simulink model "drone_PID_1126"  (R2021a)
settings: Solver=FixedStepAuto  StartTime=0.0  StopTime=10.0  RelTol=1e-3  EnableMultiTasking=on
model workspace (MAT data in the model file):
  H_G = 2
  Sv = 1300
  Ta = 4000
  Tb = 1600
  Ts = 0.016
  VOL_center = 1515
  V_G = 100
  step_R = 0.2
  volume_G = 100
undefined symbols (not defined in the file or in its folder): AUX, dev, pwm_output1
libraries: px4Sensorslib x8, cstblocks x4, px4lib x4, simulink x1, px4uORBlib x1
settings Model: ExtModeTrigDuration=10  Creator=Kawaguchi  LastModifiedBy=beket
settings SolverCC: PositivePriorityOrder=on
settings OptimizationCC: EnhancedBackFolding=on  PassReuseOutputArgsAs=Individual arguments  ZeroExternalMemoryAtStartup=off  ZeroInternalMemoryAtStartup=off  MaxStackSize=64  OptimizeBlockOrder=speed  DifferentSizesBufferReuse=on  OptimizationCustomize=off  EfficientTunableParamExpr=on
settings DebuggingCC: ParameterTunabilityLossMsg=error
settings HardwareCC: ProdBitPerPointer=32  ProdBitPerSizeT=32  ProdBitPerPtrDiffT=32  ProdLargestAtomicInteger=Long  ProdLargestAtomicFloat=Double  ProdWordSize=32  ProdLongLongMode=on  ProdHWDeviceType=ARM Compatible->ARM Cortex
settings SFSimCC: MATLABDynamicMemAlloc=off  SimTargetLang=C++
settings RTWCC: SystemTargetFile=ert.tlc  HardwareBoard=PX4 Pixhawk 4  TLCOptions="-aInlineSetEventsForThisBaseRateFcn=TLC_FALSE -aSuppressMultiTaskScheduler=TLC_FALSE  -aRateBasedStepFcn=0"  TemplateMakefile=ert_default_tmf  Toolchain=GNU Tools for PX4 Autopilots  TargetLang=C++
settings CodeAppCC: ForceParamTrailComments=on  IgnoreCustomStorageClasses=off  OperatorAnnotations=on  SimulinkDataObjDesc=on  SFDataObjDesc=on  InsertBlockDesc=on
settings ERTTargetCC: ExtModeTransport=3  ExtModeStaticAlloc=on  ExtModeStaticAllocSize=1024  ExtModeMexFile=ext_xcp  ExtModeIntrfLevel=Level2 - Open

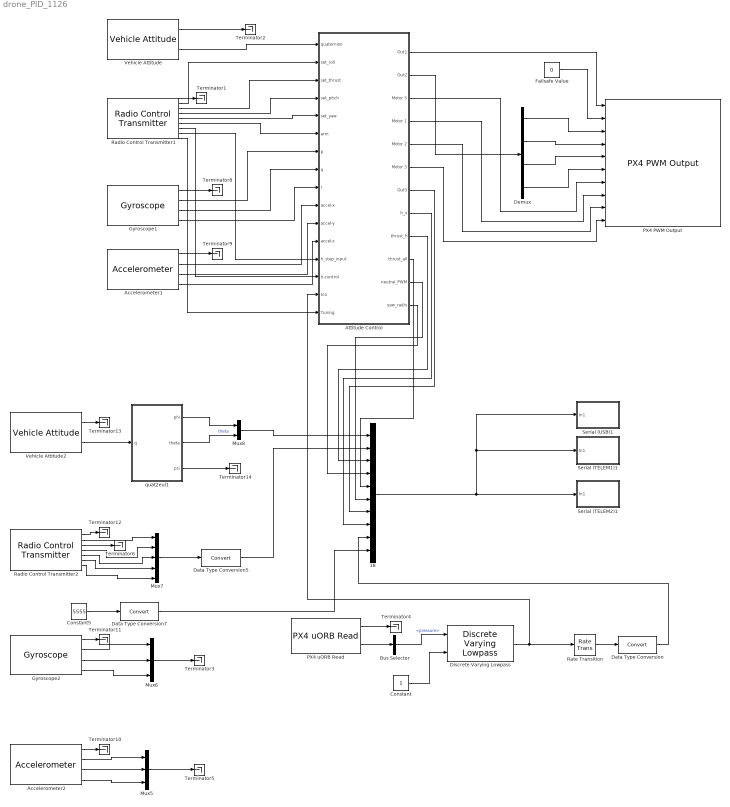
== system drone_PID_1126 ==
  18 : Mux  Inputs=10
  Accelerometer1 : px4Sensorslib/Accelerometer  uorbTimeStamp=off  BlockingMode=off  BlockTimeout=1e-3  sampleTime=1/250
      settings: SourceProductBaseCode=PX4AUTOPILOTS
  Accelerometer2 : px4Sensorslib/Accelerometer  uorbTimeStamp=off  BlockingMode=off  BlockTimeout=1e-3  sampleTime=Ts
      settings: SourceProductBaseCode=PX4AUTOPILOTS
  Attitude Control : Subsystem
  Bus Selector : BusSelector  OutputSignals=pressure
  Constant : Constant
  Constant5 : Constant  Value=5555
  Data Type Conversion : DataTypeConversion
  Data Type Conversion5 : DataTypeConversion
  Data Type Conversion7 : DataTypeConversion
  Demux : Demux
  Discrete Varying Lowpass : cstblocks/Linear Parameter Varying/Discrete Varying Lowpass  N=1  w0=0  Ts=1/250
      settings: SourceProductBaseCode=CT
  Failsafe Value : Constant  Value=0  OutDataTypeStr=boolean  SampleTime=-1
  Gyroscope1 : px4Sensorslib/Gyroscope  uorbTimeStamp=off  BlockingMode=off  BlockTimeout=1e-3  sampleTime=1/250
      settings: SourceProductBaseCode=PX4AUTOPILOTS
  Gyroscope2 : px4Sensorslib/Gyroscope  uorbTimeStamp=off  BlockingMode=off  BlockTimeout=1e-3  sampleTime=Ts
      settings: SourceProductBaseCode=PX4AUTOPILOTS
  Mux5 : Mux  Inputs=3
  Mux6 : Mux  Inputs=3
  Mux7 : Mux  Inputs=5
  Mux8 : Mux  Inputs=2
  PX4 PWM Output : px4lib/PX4 PWM Output  pwmDevice=AUX (/dev/pwm_output1)  pwmChannel1_=on  pwmChannel2_=on  pwmChannel3_=on  pwmChannel4_=on  pwmChannel5_=on  pwmChannel6_=on  pwmChannel7_=on  pwmChannel8_=on  forceTerminateFailsafe=off  outputErrorStatus=off
      settings: SourceProductBaseCode=PX4AUTOPILOTS
  PX4 uORB Read : px4uORBlib/PX4 uORB Read  uORBTopic=sensor_baro  selectInstance=sensor_baro  SampleTime=1/250  BlockingMode=off  BlockTimeout=1e-3
      settings: SourceProductBaseCode=PX4AUTOPILOTS
  Radio Control Transmitter1 : px4Sensorslib/Radio Control Transmitter  channel1=on  channel2=on  channel3=on  channel4=on  channel5=on  channel6=on  channel7=on  channel8=on  channel_count=off  rssi=off  rc_input_source=off  timestamp_last_signal=off  time_stamp=off  sampleTime=1/250  BlockingMode=off  BlockTimeout=5
      settings: SourceProductBaseCode=PX4AUTOPILOTS
  Radio Control Transmitter2 : px4Sensorslib/Radio Control Transmitter  channel1=on  channel2=on  channel3=on  channel4=on  channel5=on  channel6=off  channel7=on  channel8=off  channel_count=off  rssi=off  rc_input_source=off  timestamp_last_signal=off  time_stamp=off  sampleTime=Ts  BlockingMode=off  BlockTimeout=5
      settings: SourceProductBaseCode=PX4AUTOPILOTS
  Rate Transition : RateTransition  OutPortSampleTimeOpt=Multiple of input port sample time  OutPortSampleTimeMultiple=4  OutPortSampleTime=4
  Serial (TELEM1)1 : Subsystem
  Serial (TELEM2)1 : Subsystem
  Serial (USB)1 : Subsystem
  Terminator{1..6,8..14} (13 alike) : Terminator
  Vehicle Attitude : px4Sensorslib/Vehicle Attitude  rollRate=off  pitchRate=off  yawRate=off  quaternion=on  uorbTimeStamp=off  BlockingMode=off  BlockTimeout=0.001  sampleTime=1/250
      settings: SourceProductBaseCode=PX4AUTOPILOTS
  Vehicle Attitude2 : px4Sensorslib/Vehicle Attitude  rollRate=off  pitchRate=off  yawRate=off  quaternion=on  uorbTimeStamp=off  BlockingMode=off  BlockTimeout=0.001  sampleTime=Ts
      settings: SourceProductBaseCode=PX4AUTOPILOTS
  quat2eul1 : MATLAB Function  TreatAsAtomicUnit=on
  wires:
  Vehicle Attitude/1 -> Terminator2/1
  Vehicle Attitude/2 -> Attitude Control/1(quaternion)
  Radio Control Transmitter1/1 -> Terminator1/1
  Radio Control Transmitter1/2 -> Attitude Control/2(set_roll)
  Radio Control Transmitter1/3 -> Attitude Control/3(set_thrust)
  Radio Control Transmitter1/4 -> Attitude Control/4(set_pitch)
  Radio Control Transmitter1/5 -> Attitude Control/5(set_yaw)
  Radio Control Transmitter1/6 -> Attitude Control/6(arm)
  Accelerometer1/1 -> Terminator9/1
  Gyroscope1/1 -> Terminator8/1
  Gyroscope1/2 -> Attitude Control/7(p)
  Gyroscope1/3 -> Attitude Control/8(q)
  Gyroscope1/4 -> Attitude Control/9(r)
  Accelerometer1/2 -> Attitude Control/10(accel-x)
  Accelerometer1/3 -> Attitude Control/11(accel-y)
  Accelerometer1/4 -> Attitude Control/12(accel-z)
  Data Type Conversion7/1 -> 18/10
  Accelerometer2/4 -> Mux5/3
  quat2eul1/2(theta) -> Mux8/2  "theta"
  Radio Control Transmitter2/4 -> Mux7/2
  Mux7/1 -> Data Type Conversion5/1
  18/1 -> Serial (TELEM1)1/1(In1), Serial (USB)1/1(In1), Serial (TELEM2)1/1(In1)
  Gyroscope2/4 -> Mux6/3
  quat2eul1/1(phi) -> Mux8/1
  Radio Control Transmitter2/1 -> Terminator12/1
  Gyroscope2/1 -> Terminator11/1
  Accelerometer2/3 -> Mux5/2
  Constant5/1 -> Data Type Conversion7/1
  Accelerometer2/2 -> Mux5/1
  Radio Control Transmitter2/3 -> Terminator6/1
  Accelerometer2/1 -> Terminator10/1
  Vehicle Attitude2/1 -> Terminator13/1
  Radio Control Transmitter2/2 -> Mux7/1
  Gyroscope2/3 -> Mux6/2
  quat2eul1/3(psi) -> Terminator14/1
  Gyroscope2/2 -> Mux6/1
  Vehicle Attitude2/2 -> quat2eul1/1(q)
  Mux8/1 -> 18/1
  Data Type Conversion5/1 -> 18/2
  Mux5/1 -> Terminator5/1
  Attitude Control/1(Out1) -> PX4 PWM Output/1
  Demux/1 -> PX4 PWM Output/3
  Demux/2 -> PX4 PWM Output/4
  Demux/3 -> PX4 PWM Output/5
  Demux/4 -> PX4 PWM Output/6
  Failsafe Value/1 -> PX4 PWM Output/2
  Attitude Control/3(Motor 5) -> PX4 PWM Output/7
  Attitude Control/4(Motor 1) -> PX4 PWM Output/8
  Attitude Control/5(Motor 2) -> PX4 PWM Output/9
  Attitude Control/6(Motor 3) -> PX4 PWM Output/10
  Radio Control Transmitter2/5 -> Mux7/3
  Attitude Control/7(Out3) -> 18/7
  Mux6/1 -> Terminator3/1
  Radio Control Transmitter2/6 -> Mux7/4
  PX4 uORB Read/1 -> Terminator4/1
  PX4 uORB Read/2 -> Bus Selector/1
  Bus Selector/1 -> Discrete Varying Lowpass/1  "<pressure>"
  Data Type Conversion/1 -> 18/9
  Discrete Varying Lowpass/1 -> Rate Transition/1, Attitude Control/15(In1)
  Constant/1 -> Discrete Varying Lowpass/2
  Radio Control Transmitter2/7 -> Mux7/5
  Radio Control Transmitter1/8 -> Attitude Control/13(h_step_input)
  Radio Control Transmitter1/7 -> Attitude Control/14(h-control)
  Rate Transition/1 -> Data Type Conversion/1
  Radio Control Transmitter1/9 -> Attitude Control/16(Tuning)
  Attitude Control/8(h_x) -> 18/8
  Attitude Control/2(Out2) -> Demux/1
  Attitude Control/9(thrust_h) -> 18/3
  Attitude Control/12(yaw_rad/s) -> 18/4
  Attitude Control/10(thrust_all) -> 18/5
  Attitude Control/11(neutral_PWM) -> 18/6

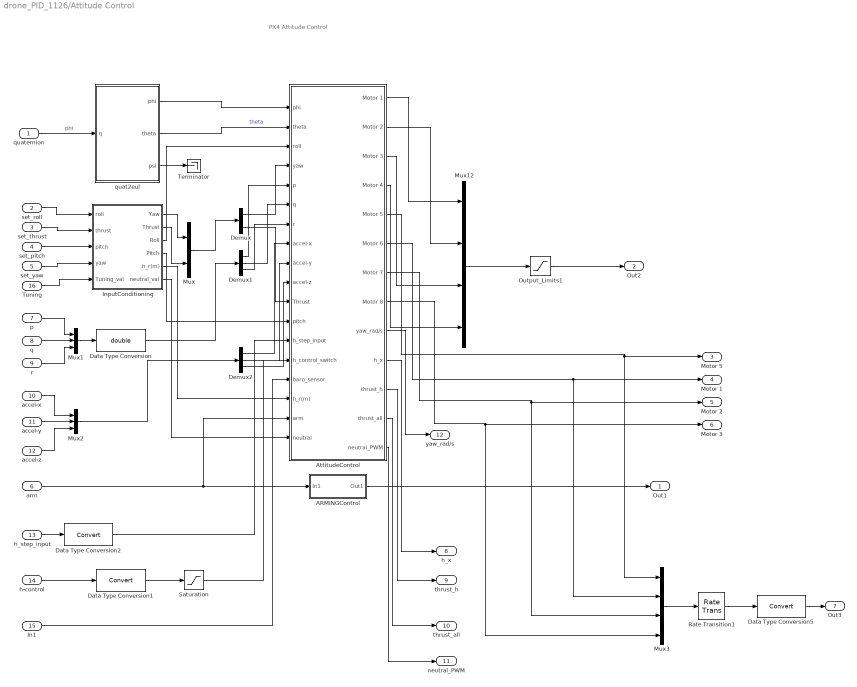
== system drone_PID_1126/Attitude Control ==
  note: PX4 Attitude Control
  quaternion : Inport
  set_roll : Inport  Port=2  OutDataTypeStr=uint16
  set_thrust : Inport  Port=3  OutDataTypeStr=uint16
  set_pitch : Inport  Port=4  OutDataTypeStr=uint16
  set_yaw : Inport  Port=5  OutDataTypeStr=uint16
  arm : Inport  Port=6  OutDataTypeStr=uint16
  p : Inport  Port=7
  q : Inport  Port=8
  r : Inport  Port=9
  accel-x : Inport  Port=10
  accel-y : Inport  Port=11
  accel-z : Inport  Port=12
  h_step_input : Inport  Port=13
  h-control : Inport  Port=14
  In1 : Inport  Port=15
  Tuning : Inport  Port=16
  ARMINGControl : Subsystem
  AttitudeControl : Subsystem
  Data Type Conversion : DataTypeConversion  OutDataTypeStr=double
  Data Type Conversion1 : DataTypeConversion
  Data Type Conversion2 : DataTypeConversion
  Data Type Conversion5 : DataTypeConversion
  Demux : Demux  Outputs=2
  Demux1 : Demux  Outputs=3
  Demux2 : Demux  Outputs=3
  InputConditioning : Subsystem
  Mux : Mux  Inputs=2
  Mux1 : Mux  Inputs=3
  Mux12 : Mux
  Mux2 : Mux  Inputs=3
  Mux3 : Mux
  Output_Limits1 : Saturate  UpperLimit=2000  LowerLimit=1000
  Rate Transition1 : RateTransition  OutPortSampleTimeOpt=Multiple of input port sample time  OutPortSampleTimeMultiple=4
  Saturation : Saturate  UpperLimit=1600  LowerLimit=0
  Terminator : Terminator
  quat2eul : MATLAB Function  TreatAsAtomicUnit=on
  Out1 : Outport  VectorParamsAs1DForOutWhenUnconnected=off
  Out2 : Outport  Port=2  VectorParamsAs1DForOutWhenUnconnected=off
  Motor 5 : Outport  Port=3  OutDataTypeStr=uint16  VectorParamsAs1DForOutWhenUnconnected=off
  Motor 1 : Outport  Port=4  OutDataTypeStr=uint16  VectorParamsAs1DForOutWhenUnconnected=off
  Motor 2 : Outport  Port=5  OutDataTypeStr=uint16  VectorParamsAs1DForOutWhenUnconnected=off
  Motor 3 : Outport  Port=6  OutDataTypeStr=uint16  VectorParamsAs1DForOutWhenUnconnected=off
  Out3 : Outport  Port=7
  h_x : Outport  Port=8
  thrust_h : Outport  Port=9
  thrust_all : Outport  Port=10
  neutral_PWM : Outport  Port=11
  yaw_rad/s : Outport  Port=12
  wires:
  set_roll/1 -> InputConditioning/1(roll)
  arm/1 -> AttitudeControl/17(arm), ARMINGControl/1(In1)
  quat2eul/2(theta) -> AttitudeControl/2(theta)  "theta"
  Output_Limits1/1 -> Out2/1
  Mux12/1 -> Output_Limits1/1
  ARMINGControl/1(Out1) -> Out1/1
  set_yaw/1 -> InputConditioning/4(yaw)
  quaternion/1 -> quat2eul/1(q)  "phi"
  quat2eul/1(phi) -> AttitudeControl/1(phi)
  quat2eul/3(psi) -> Terminator/1
  AttitudeControl/1(Motor 1) -> Mux12/1
  AttitudeControl/2(Motor 2) -> Mux12/2
  AttitudeControl/3(Motor 3) -> Mux12/3
  AttitudeControl/4(Motor 4) -> Mux12/4
  Mux/1 -> Demux/1
  p/1 -> Mux1/1
  r/1 -> Mux1/3
  Mux1/1 -> Data Type Conversion/1
  Demux1/2 -> AttitudeControl/6(q)
  Demux1/1 -> AttitudeControl/5(p)
  Demux1/3 -> AttitudeControl/7(r)
  accel-y/1 -> Mux2/2
  accel-x/1 -> Mux2/1
  accel-z/1 -> Mux2/3
  Mux2/1 -> Demux2/1
  Demux2/2 -> AttitudeControl/9(accel-y)
  Demux2/1 -> AttitudeControl/8(accel-x)
  Demux2/3 -> AttitudeControl/10(accel-z)
  InputConditioning/1(Yaw) -> Mux/1
  InputConditioning/2(Thrust) -> Mux/2
  Demux/1 -> AttitudeControl/4(yaw)
  Demux/2 -> AttitudeControl/11(Thrust)
  InputConditioning/3(Roll) -> AttitudeControl/3(roll)
  InputConditioning/4(Pitch) -> AttitudeControl/12(pitch)
  set_thrust/1 -> InputConditioning/2(thrust)
  set_pitch/1 -> InputConditioning/3(pitch)
  q/1 -> Mux1/2
  Data Type Conversion/1 -> Demux1/1
  AttitudeControl/5(Motor 5) -> Mux3/1, Motor 5/1
  AttitudeControl/8(Motor 8) -> Mux3/4, Motor 3/1
  AttitudeControl/7(Motor 7) -> Mux3/3, Motor 2/1
  AttitudeControl/6(Motor 6) -> Mux3/2, Motor 1/1
  Mux3/1 -> Rate Transition1/1
  Data Type Conversion5/1 -> Out3/1
  Rate Transition1/1 -> Data Type Conversion5/1
  AttitudeControl/9(yaw_rad/s) -> yaw_rad/s/1
  h_step_input/1 -> Data Type Conversion2/1
  Data Type Conversion2/1 -> AttitudeControl/13(h_step_input)
  h-control/1 -> Data Type Conversion1/1
  Data Type Conversion1/1 -> Saturation/1
  In1/1 -> AttitudeControl/15(baro_sensor)
  AttitudeControl/10(h_x) -> h_x/1
  InputConditioning/5(h_r(m)) -> AttitudeControl/16(h_r(m))
  Tuning/1 -> InputConditioning/5(Tuning_val)
  InputConditioning/6(neutral_val) -> AttitudeControl/18(neutral)
  Saturation/1 -> AttitudeControl/14(h_control_switch)
  AttitudeControl/11(thrust_h) -> thrust_h/1
  AttitudeControl/12(thrust_all) -> thrust_all/1
  AttitudeControl/13(neutral_PWM) -> neutral_PWM/1

== system drone_PID_1126/Serial (TELEM1)1 ==
  In1 : Inport
  Cast To Single1 : DataTypeConversion  OutDataTypeStr=single
  Serial Transmit1 : px4lib/Serial Transmit  SCIModule=/dev/ttyS1
      settings: SourceProductBaseCode=PX4AUTOPILOTS
  wires:
  Cast To Single1/1 -> Serial Transmit1/1
  In1/1 -> Cast To Single1/1

== system drone_PID_1126/Serial (TELEM2)1 ==
  In1 : Inport
  Cast To Single1 : DataTypeConversion  OutDataTypeStr=single
  Serial Transmit1 : px4lib/Serial Transmit  SCIModule=/dev/ttyS2
      settings: SourceProductBaseCode=PX4AUTOPILOTS
  wires:
  Cast To Single1/1 -> Serial Transmit1/1
  In1/1 -> Cast To Single1/1

== system drone_PID_1126/Serial (USB)1 ==
  In1 : Inport
  Cast To Single1 : DataTypeConversion  OutDataTypeStr=single
  Serial Transmit1 : px4lib/Serial Transmit  SCIModule=/dev/ttyACM0
      settings: SourceProductBaseCode=PX4AUTOPILOTS
  wires:
  Cast To Single1/1 -> Serial Transmit1/1
  In1/1 -> Cast To Single1/1

== system drone_PID_1126/Attitude Control/ARMINGControl ==
  In1 : Inport
  Compare To Constant3 : simulink/Logic and Bit Operations/Compare To Constant  relop=>=  const=uint16(1500)  OutDataTypeStr=boolean
  Out1 : Outport  VectorParamsAs1DForOutWhenUnconnected=off
  wires:
  Compare To Constant3/1 -> Out1/1
  In1/1 -> Compare To Constant3/1

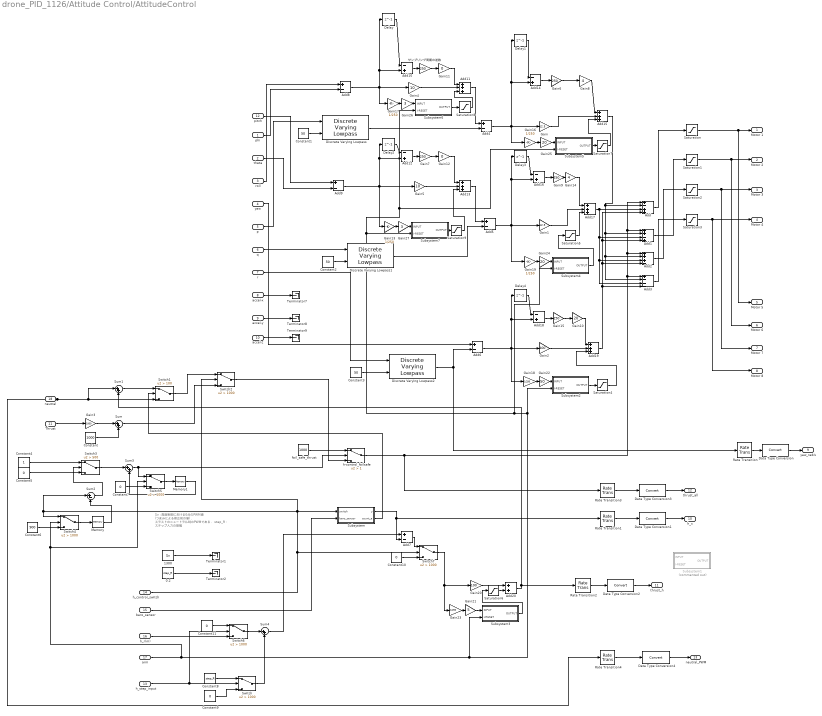
== system drone_PID_1126/Attitude Control/AttitudeControl ==
  note: Sv : 高度制御における0点のPWM値
      | 	(つまみによる修正前の値)．
      | スラストのニュートラル時のPWMである．
      |
      | step_R : ステップ入力の振幅
  phi : Inport
  theta : Inport  Port=2
  roll : Inport  Port=3
  yaw : Inport  Port=4
  p : Inport  Port=5
  q : Inport  Port=6
  r : Inport  Port=7
  accel-x : Inport  Port=8
  accel-y : Inport  Port=9
  accel-z : Inport  Port=10
  Thrust : Inport  Port=11
  pitch : Inport  Port=12
  h_step_input : Inport  Port=13
  h_control_switch : Inport  Port=14
  baro_sensor : Inport  Port=15
  h_r(m) : Inport  Port=16
  arm : Inport  Port=17
  neutral : Inport  Port=18
  0.2 : Constant  Value=step_R
  1300 : Constant  Value=Sv
  Add : Sum  Inputs=+-++
  Add1 : Sum  Inputs=++-+
  Add{10,12,14,16,18} (5 alike) : Sum  Inputs=-+
  Add{11,13,15,17,19} (5 alike) : Sum  Inputs=+++
  Add2 : Sum  Inputs=+++-
  Add20 : Sum
  Add3 : Sum  Inputs=+---
  Add{4..9} (6 alike) : Sum  Inputs=+-
  Constant : Constant  Value=1000
  Constant1 : Constant  Value=50
  Constant{5,7,9..11} (5 alike) : Constant  Value=0
  Constant2 : Constant  Value=50
  Constant3 : Constant  Value=50
  Constant4 : Constant
  Constant6 : Constant  Value=900
  Constant8 : Constant  Value=step_R
  Data Type Conversion{,1..4} (5 alike) : DataTypeConversion
  Delay{,1..4} (5 alike) : Delay  DelayLength=1  InitialCondition=0
  Discrete Varying Lowpass : cstblocks/Linear Parameter Varying/Discrete Varying Lowpass  N=1  w0=0  Ts=1/250
      settings: SourceProductBaseCode=CT
  Discrete Varying Lowpass1 : cstblocks/Linear Parameter Varying/Discrete Varying Lowpass  N=1  w0=0  Ts=1/250
      settings: SourceProductBaseCode=CT
  Discrete Varying Lowpass2 : cstblocks/Linear Parameter Varying/Discrete Varying Lowpass  N=1  w0=0  Ts=1/250
      settings: SourceProductBaseCode=CT
  Gain : Gain  Gain=12.5
  Gain1 : Gain  Gain=12.5
  Gain10 : Gain  Gain=20
  Gain11 : Gain  Gain=0
  Gain12 : Gain  Gain=0
  Gain{13,16..19,23} (6 alike) : Gain  Gain=1/250
  Gain14 : Gain  Gain=4
  Gain{6..7,9,15} (4 alike) : Gain  Gain=250
  Gain2 : Gain  Gain=400
  Gain20 : Gain  Gain=100
  Gain21 : Gain  Gain=5
  Gain22 : Gain  Gain=50
  Gain24 : Gain  Gain=20
  Gain25 : Gain  Gain=20
  Gain26 : Gain  Gain=3
  Gain27 : Gain  Gain=3
  Gain3 : Gain  Gain=1000
  Gain4 : Gain  Gain=10
  Gain5 : Gain  Gain=10
  Gain8 : Gain  Gain=4
  Memory : Memory  InitialCondition=900  InheritSampleTime=on
  Memory1 : Memory  InheritSampleTime=on
  Rate Transition{,1..4} (5 alike) : RateTransition  OutPortSampleTimeOpt=Multiple of input port sample time  OutPortSampleTimeMultiple=4  OutPortSampleTime=4
  Saturation{,1..3} (4 alike) : Saturate  UpperLimit=2000  LowerLimit=1000  OutDataTypeStr=uint16
  Saturation{4..5,7..9} (5 alike) : Saturate  UpperLimit=100  LowerLimit=-100
  Saturation6 : Saturate  UpperLimit=50  LowerLimit=-50
  Subsystem : Subsystem
  Subsystem1 : Subsystem  Commented=on
  Subsystem2 : Subsystem
  Subsystem3 : Subsystem
  Subsystem4 : Subsystem
  Subsystem5 : Subsystem
  Subsystem6 : Subsystem
  Subsystem7 : Subsystem
  Sum{,1,3..4} (4 alike) : Sum  Inputs=|++
  Sum2 : Sum  Inputs=|+-
  Switch{,2,4..7} (6 alike) : Switch  Criteria=u2 > Threshold  Threshold=1000
  Switch1 : Switch  Criteria=u2 > Threshold  Threshold=100
  Switch3 : Switch  Criteria=u2 > Threshold  Threshold=500
  Terminator{1..2,7..9} (5 alike) : Terminator
  fail_safe_thrust : Constant  Value=1000
  h-control_failsafe : Switch  Criteria=u2 > Threshold  Threshold=1
  サンプリング周期の逆数 : Gain  Gain=250
  Motor 1 : Outport  OutDataTypeStr=uint16  VectorParamsAs1DForOutWhenUnconnected=off
  Motor 2 : Outport  Port=2  OutDataTypeStr=uint16  VectorParamsAs1DForOutWhenUnconnected=off
  Motor 3 : Outport  Port=3  OutDataTypeStr=uint16  VectorParamsAs1DForOutWhenUnconnected=off
  Motor 4 : Outport  Port=4  OutDataTypeStr=uint16  VectorParamsAs1DForOutWhenUnconnected=off
  Motor 5 : Outport  Port=5  OutDataTypeStr=uint16  SampleTime=1/250  VectorParamsAs1DForOutWhenUnconnected=off
  Motor 6 : Outport  Port=6  OutDataTypeStr=uint16  VectorParamsAs1DForOutWhenUnconnected=off
  Motor 7 : Outport  Port=7  OutDataTypeStr=uint16  VectorParamsAs1DForOutWhenUnconnected=off
  Motor 8 : Outport  Port=8  OutDataTypeStr=uint16  VectorParamsAs1DForOutWhenUnconnected=off
  yaw_rad/s : Outport  Port=9
  h_x : Outport  Port=10
  thrust_h : Outport  Port=11
  thrust_all : Outport  Port=12
  neutral_PWM : Outport  Port=13
  wires:
  Add2/1 -> Saturation2/1
  Gain/1 -> Add15/2
  Add17/1 -> Add2/3, Add3/3, Add1/3, Add/3
  Add18/1 -> Gain15/1
  Add13/1 -> Add5/1
  Add14/1 -> Gain6/1
  Gain15/1 -> Gain10/1
  Gain11/1 -> Add11/1
  Gain1/1 -> Add17/2
  theta/1 -> Add9/2
  Gain14/1 -> Add17/1
  Gain12/1 -> Add13/1
  Gain5/1 -> Add13/2
  Saturation/1 -> Motor 5/1, Motor 1/1
  r/1 -> Discrete Varying Lowpass2/1
  Gain9/1 -> Gain14/1
  Gain6/1 -> Gain8/1
  Gain7/1 -> Gain12/1
  Add19/1 -> Add2/4, Add1/4, Add/4, Add3/4
  Add15/1 -> Add/2, Add1/2, Add2/2, Add3/2
  Add16/1 -> Gain9/1
  accel-z/1 -> Terminator9/1
  Delay3/1 -> Add16/1
  Gain10/1 -> Add19/1
  Delay/1 -> Add10/1
  Gain4/1 -> Add11/2
  サンプリング周期の逆数/1 -> Gain11/1
  Delay4/1 -> Add18/1
  Delay2/1 -> Add12/1
  Add11/1 -> Add4/1
  Add12/1 -> Gain7/1
  accel-x/1 -> Terminator7/1
  Add3/1 -> Saturation3/1
  Gain2/1 -> Add19/2
  Saturation2/1 -> Motor 7/1, Motor 3/1
  Add/1 -> Saturation/1
  Add10/1 -> サンプリング周期の逆数/1
  roll/1 -> Add8/1
  phi/1 -> Add8/2
  pitch/1 -> Add9/1
  Saturation3/1 -> Motor 8/1, Motor 4/1
  Add1/1 -> Saturation1/1
  accel-y/1 -> Terminator8/1
  Saturation1/1 -> Motor 6/1, Motor 2/1
  p/1 -> Discrete Varying Lowpass/1
  q/1 -> Discrete Varying Lowpass1/1
  Gain8/1 -> Add15/1
  yaw/1 -> Add6/1
  Delay1/1 -> Add14/1
  Subsystem6/1(OUTPUT) -> Saturation8/1
  Subsystem7/1(OUTPUT) -> Saturation9/1
  Add4/1 -> Gain16/1, Gain/1, Add14/2, Delay1/1
  Subsystem2/1(OUTPUT) -> Saturation4/1
  Discrete Varying Lowpass/1 -> Add4/2
  Constant1/1 -> Discrete Varying Lowpass/2
  Discrete Varying Lowpass1/1 -> Add5/2
  Constant2/1 -> Discrete Varying Lowpass1/2
  Constant3/1 -> Discrete Varying Lowpass2/2
  Discrete Varying Lowpass2/1 -> Rate Transition/1, Add6/2
  Rate Transition/1 -> Data Type Conversion/1
  Data Type Conversion/1 -> yaw_rad/s/1
  Add8/1 -> Gain17/1, Gain4/1, Delay/1, Add10/2
  Add6/1 -> Delay4/1, Add18/2, Gain2/1, Gain18/1
  Add9/1 -> Delay2/1, Add12/2, Gain13/1, Gain5/1
  Add5/1 -> Delay3/1, Add16/2, Gain1/1, Gain19/1
  1300/1 -> Terminator1/1
  Constant/1 -> Sum/2
  neutral/1 -> Sum1/1, Switch1/3, Rate Transition4/1
  Thrust/1 -> Gain3/1
  Gain3/1 -> Sum/1
  Rate Transition1/1 -> Data Type Conversion1/1
  Data Type Conversion1/1 -> h_x/1
  Subsystem/1(y) -> Rate Transition1/1, Add7/2
  baro_sensor/1 -> Subsystem/2(baro_sensor)
  Sum/1 -> Switch2/3
  h-control_failsafe/1 -> Rate Transition3/1, Add3/1, Add/1, Add1/1, Add2/1
  Gain21/1 -> Subsystem3/1(INPUT)
  Add7/1 -> Switch7/1
  Sum4/1 -> Add7/1
  Gain20/1 -> Add20/1
  Add20/1 -> Rate Transition2/1, Sum1/2
  Subsystem3/1(OUTPUT) -> Saturation6/1
  Switch7/1 -> Gain23/1, Gain20/1
  Constant10/1 -> Switch7/3
  arm/1 -> Switch5/2, Switch4/2, Subsystem3/2(I-RESET), Subsystem5/2(I-RESET), Subsystem6/2(I-RESET), Subsystem7/2(I-RESET), Subsystem4/2(I-RESET), Subsystem2/2(I-RESET)
  Gain22/1 -> Subsystem2/1(INPUT)
  Gain18/1 -> Gain22/1
  h_control_switch/1 -> Sum2/1, Switch4/1, Switch2/2, Subsystem/1(switch), Switch7/2
  Gain23/1 -> Gain21/1
  Saturation4/1 -> Add19/3
  Gain19/1 -> Gain24/1
  Gain24/1 -> Subsystem4/1(INPUT)
  Subsystem4/1(OUTPUT) -> Saturation5/1
  Saturation5/1 -> Add17/3
  Saturation6/1 -> Add20/2
  Gain25/1 -> Subsystem5/1(INPUT)
  Gain16/1 -> Gain25/1
  Gain17/1 -> Gain26/1
  Gain26/1 -> Subsystem6/1(INPUT)
  Gain27/1 -> Subsystem7/1(INPUT)
  Gain13/1 -> Gain27/1
  Subsystem5/1(OUTPUT) -> Saturation7/1
  Saturation7/1 -> Add15/3
  Saturation8/1 -> Add11/3
  Saturation9/1 -> Add13/3
  Subsystem/2(count_a) -> Switch1/2
  Sum1/1 -> Switch1/1
  Switch1/1 -> Switch2/1
  Constant4/1 -> Switch3/1
  Constant5/1 -> Switch3/3
  Memory/1 -> Sum2/2
  Sum2/1 -> Switch3/2
  Switch3/1 -> Sum3/1
  Sum3/1 -> Switch5/1, h-control_failsafe/2
  Memory1/1 -> Sum3/2
  fail_safe_thrust/1 -> h-control_failsafe/1
  Switch4/1 -> Memory/1
  Constant6/1 -> Switch4/3
  Switch5/1 -> Memory1/1
  Constant7/1 -> Switch5/3
  Switch2/1 -> h-control_failsafe/3
  h_step_input/1 -> Switch6/2, Switch/2
  Constant8/1 -> Switch/1
  Constant9/1 -> Switch/3
  h_r(m)/1 -> Switch6/3
  Switch/1 -> Sum4/2
  Switch6/1 -> Sum4/1
  Constant11/1 -> Switch6/1
  0.2/1 -> Terminator2/1
  Rate Transition2/1 -> Data Type Conversion2/1
  Data Type Conversion2/1 -> thrust_h/1
  Rate Transition3/1 -> Data Type Conversion3/1
  Data Type Conversion3/1 -> thrust_all/1
  Rate Transition4/1 -> Data Type Conversion4/1
  Data Type Conversion4/1 -> neutral_PWM/1

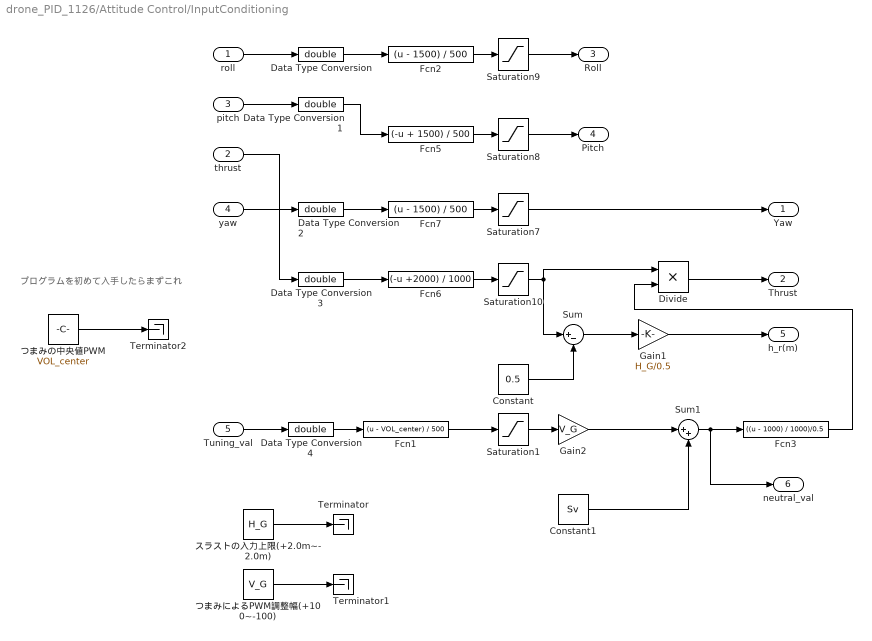
== system drone_PID_1126/Attitude Control/InputConditioning ==
  note: プログラムを初めて入手したらまずこれ
  roll : Inport
  thrust : Inport  Port=2
  pitch : Inport  Port=3
  yaw : Inport  Port=4
  Tuning_val : Inport  Port=5
  Constant : Constant  Value=0.5
  Constant1 : Constant  Value=Sv
  Data Type Conversion{,1..4} (5 alike) : DataTypeConversion  OutDataTypeStr=double
  Divide : Product  Inputs=**
  Fcn1 : Fcn  Expr=(u - VOL_center) / 500
  Fcn2 : Fcn  Expr=(u - 1500) / 500
  Fcn3 : Fcn  Expr=((u - 1000) / 1000)/0.5
  Fcn5 : Fcn  Expr=(-u + 1500) / 500
  Fcn6 : Fcn  Expr=(-u +2000) / 1000
  Fcn7 : Fcn  Expr=(u - 1500) / 500
  Gain1 : Gain  Gain=H_G/0.5
  Gain2 : Gain  Gain=V_G
  Saturation{1,7..9} (4 alike) : Saturate  UpperLimit=1  LowerLimit=-1
  Saturation10 : Saturate  UpperLimit=1  LowerLimit=0
  Sum : Sum  Inputs=|+-
  Sum1 : Sum  Inputs=|++
  Terminator : Terminator
  Terminator1 : Terminator
  Terminator2 : Terminator
  つまみによるPWM調整幅(+100~-100) : Constant  Value=V_G
  つまみの中央値PWM : Constant  Value=VOL_center
  スラストの入力上限(+2.0m~-2.0m) : Constant  Value=H_G
  Yaw : Outport  VectorParamsAs1DForOutWhenUnconnected=off
  Thrust : Outport  Port=2  VectorParamsAs1DForOutWhenUnconnected=off
  Roll : Outport  Port=3  VectorParamsAs1DForOutWhenUnconnected=off
  Pitch : Outport  Port=4  VectorParamsAs1DForOutWhenUnconnected=off
  h_r(m) : Outport  Port=5
  neutral_val : Outport  Port=6
  wires:
  Saturation10/1 -> Divide/1, Sum/1
  Saturation7/1 -> Yaw/1
  Saturation8/1 -> Pitch/1
  Fcn6/1 -> Saturation10/1
  thrust/1 -> Data Type Conversion3/1
  Fcn2/1 -> Saturation9/1
  Fcn5/1 -> Saturation8/1
  Saturation9/1 -> Roll/1
  Fcn7/1 -> Saturation7/1
  yaw/1 -> Data Type Conversion2/1
  pitch/1 -> Data Type Conversion1/1
  roll/1 -> Data Type Conversion/1
  Data Type Conversion/1 -> Fcn2/1
  Data Type Conversion1/1 -> Fcn5/1
  Data Type Conversion2/1 -> Fcn7/1
  Data Type Conversion3/1 -> Fcn6/1
  Divide/1 -> Thrust/1
  Constant/1 -> Sum/2
  Sum/1 -> Gain1/1
  Gain1/1 -> h_r(m)/1
  スラストの入力上限(+2.0m~-2.0m)/1 -> Terminator/1
  Tuning_val/1 -> Data Type Conversion4/1
  Fcn1/1 -> Saturation1/1
  Saturation1/1 -> Gain2/1
  Data Type Conversion4/1 -> Fcn1/1
  Gain2/1 -> Sum1/1
  Sum1/1 -> neutral_val/1, Fcn3/1
  Constant1/1 -> Sum1/2
  Fcn3/1 -> Divide/2
  つまみによるPWM調整幅(+100~-100)/1 -> Terminator1/1
  つまみの中央値PWM/1 -> Terminator2/1

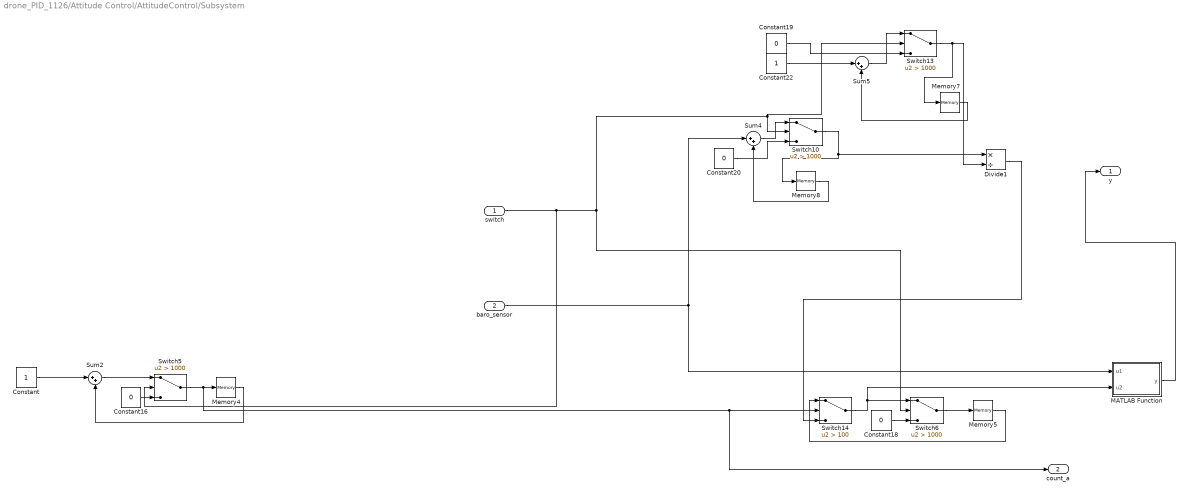
== system drone_PID_1126/Attitude Control/AttitudeControl/Subsystem ==
  switch : Inport
  baro_sensor : Inport  Port=2
  Constant : Constant
  Constant{16,18..20} (4 alike) : Constant  Value=0
  Constant22 : Constant
  Divide1 : Product  Inputs=*/
  MATLAB Function : MATLAB Function  TreatAsAtomicUnit=on
  Memory{4..5,7..8} (4 alike) : Memory  InheritSampleTime=on
  Sum2 : Sum  Inputs=|++
  Sum4 : Sum  Inputs=|++
  Sum5 : Sum  Inputs=|++
  Switch{5..6,10,13} (4 alike) : Switch  Criteria=u2 > Threshold  Threshold=1000
  Switch14 : Switch  Criteria=u2 > Threshold  Threshold=100
  y : Outport
  count_a : Outport  Port=2
  wires:
  Switch10/1 -> Divide1/1, Memory8/1
  switch/1 -> Switch5/2, Switch13/2, Switch10/2, Switch6/2
  Constant22/1 -> Sum5/1
  Sum5/1 -> Switch13/1
  Sum4/1 -> Switch10/1
  Constant19/1 -> Switch13/3
  Switch5/1 -> count_a/1, Switch14/2, Memory4/1
  Constant20/1 -> Switch10/3
  baro_sensor/1 -> Sum4/1, MATLAB Function/1(u1)
  Memory8/1 -> Sum4/2
  Memory7/1 -> Sum5/2
  MATLAB Function/1(y) -> y/1
  Constant18/1 -> Switch6/3
  Switch13/1 -> Divide1/2, Memory7/1
  Switch14/1 -> MATLAB Function/2(u2), Switch6/1
  Divide1/1 -> Switch14/3
  Switch6/1 -> Memory5/1
  Memory5/1 -> Switch14/1
  Memory4/1 -> Sum2/2
  Constant/1 -> Sum2/1
  Constant16/1 -> Switch5/3
  Sum2/1 -> Switch5/1

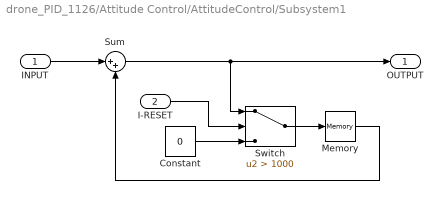
== system drone_PID_1126/Attitude Control/AttitudeControl/Subsystem1 ==
  INPUT : Inport
  I-RESET : Inport  Port=2
  Constant : Constant  Value=0
  Memory : Memory
  Sum : Sum  Inputs=|++
  Switch : Switch  Criteria=u2 > Threshold  Threshold=1000
  OUTPUT : Outport
  wires:
  I-RESET/1 -> Switch/2
  Constant/1 -> Switch/3
  INPUT/1 -> Sum/1
  Sum/1 -> OUTPUT/1, Switch/1
  Switch/1 -> Memory/1
  Memory/1 -> Sum/2

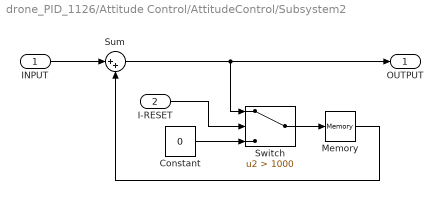
== system drone_PID_1126/Attitude Control/AttitudeControl/Subsystem2 ==
  INPUT : Inport
  I-RESET : Inport  Port=2
  Constant : Constant  Value=0
  Memory : Memory  InheritSampleTime=on
  Sum : Sum  Inputs=|++
  Switch : Switch  Criteria=u2 > Threshold  Threshold=1000
  OUTPUT : Outport
  wires:
  Memory/1 -> Sum/2
  Switch/1 -> Memory/1
  Sum/1 -> Switch/1, OUTPUT/1
  INPUT/1 -> Sum/1
  Constant/1 -> Switch/3
  I-RESET/1 -> Switch/2

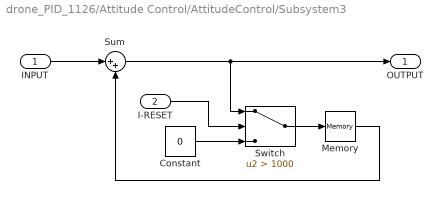
== system drone_PID_1126/Attitude Control/AttitudeControl/Subsystem3 ==
  INPUT : Inport
  I-RESET : Inport  Port=2
  Constant : Constant  Value=0
  Memory : Memory  InheritSampleTime=on
  Sum : Sum  Inputs=|++
  Switch : Switch  Criteria=u2 > Threshold  Threshold=1000
  OUTPUT : Outport
  wires:
  I-RESET/1 -> Switch/2
  Constant/1 -> Switch/3
  INPUT/1 -> Sum/1
  Sum/1 -> OUTPUT/1, Switch/1
  Switch/1 -> Memory/1
  Memory/1 -> Sum/2

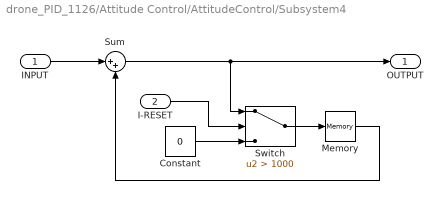
== system drone_PID_1126/Attitude Control/AttitudeControl/Subsystem4 ==
  INPUT : Inport
  I-RESET : Inport  Port=2
  Constant : Constant  Value=0
  Memory : Memory  InheritSampleTime=on
  Sum : Sum  Inputs=|++
  Switch : Switch  Criteria=u2 > Threshold  Threshold=1000
  OUTPUT : Outport
  wires:
  I-RESET/1 -> Switch/2
  Constant/1 -> Switch/3
  INPUT/1 -> Sum/1
  Sum/1 -> OUTPUT/1, Switch/1
  Switch/1 -> Memory/1
  Memory/1 -> Sum/2

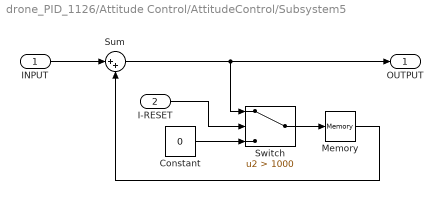
== system drone_PID_1126/Attitude Control/AttitudeControl/Subsystem5 ==
  INPUT : Inport
  I-RESET : Inport  Port=2
  Constant : Constant  Value=0
  Memory : Memory  InheritSampleTime=on
  Sum : Sum  Inputs=|++
  Switch : Switch  Criteria=u2 > Threshold  Threshold=1000
  OUTPUT : Outport
  wires:
  Memory/1 -> Sum/2
  Switch/1 -> Memory/1
  Sum/1 -> Switch/1, OUTPUT/1
  INPUT/1 -> Sum/1
  Constant/1 -> Switch/3
  I-RESET/1 -> Switch/2

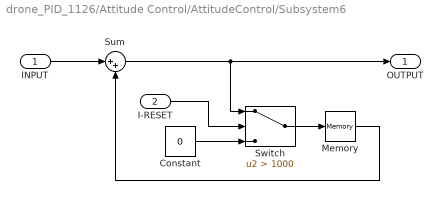
== system drone_PID_1126/Attitude Control/AttitudeControl/Subsystem6 ==
  INPUT : Inport
  I-RESET : Inport  Port=2
  Constant : Constant  Value=0
  Memory : Memory  InheritSampleTime=on
  Sum : Sum  Inputs=|++
  Switch : Switch  Criteria=u2 > Threshold  Threshold=1000
  OUTPUT : Outport
  wires:
  I-RESET/1 -> Switch/2
  Constant/1 -> Switch/3
  INPUT/1 -> Sum/1
  Sum/1 -> OUTPUT/1, Switch/1
  Switch/1 -> Memory/1
  Memory/1 -> Sum/2

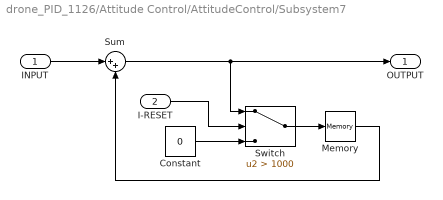
== system drone_PID_1126/Attitude Control/AttitudeControl/Subsystem7 ==
  INPUT : Inport
  I-RESET : Inport  Port=2
  Constant : Constant  Value=0
  Memory : Memory  InheritSampleTime=on
  Sum : Sum  Inputs=|++
  Switch : Switch  Criteria=u2 > Threshold  Threshold=1000
  OUTPUT : Outport
  wires:
  Memory/1 -> Sum/2
  Switch/1 -> Memory/1
  Sum/1 -> Switch/1, OUTPUT/1
  INPUT/1 -> Sum/1
  Constant/1 -> Switch/3
  I-RESET/1 -> Switch/2

== matlab function drone_PID_1126/quat2eul1 ==
  data: q input; phi output; theta output; psi output
function [phi,theta,psi] = quat2eul(q)

% Quaternion conversion to Euler angles based on the PX4 Firmware v1.6.5
% release.

phi = atan2(2*(q(1)*q(2) + q(3)* q(4)), q(1)^2 - q(2)^2 - q(3)^2 + q(4)^2);
theta = asin(-2*(q(2)*q(4) - q(1)*q(3)));
psi = atan2(2*(q(2)*q(3) + q(1)* q(4)), q(1)^2 + q(2)^2 - q(3)^2 - q(4)^2);

end

== matlab function drone_PID_1126/Attitude Control/quat2eul ==
  data: q input; phi output; theta output; psi output
function [phi,theta,psi] = quat2eul(q)

% Quaternion conversion to Euler angles based on the PX4 Firmware v1.6.5
% release.

phi = atan2(2*(q(1)*q(2) + q(3)* q(4)), q(1)^2 - q(2)^2 - q(3)^2 + q(4)^2);
theta = asin(-2*(q(2)*q(4) - q(1)*q(3)));
psi = atan2(2*(q(2)*q(3) + q(1)* q(4)), q(1)^2 + q(2)^2 - q(3)^2 - q(4)^2);

end

== matlab function drone_PID_1126/Attitude Control/AttitudeControl/Subsystem/MATLAB Function ==
  data: u1 input; y output; u2 input
function y = fcn(u1,u2)
   %気圧センサ校正部分
   q = -0.105;%高さ0.9mへの移動での気圧変化(hPa)
   qq = 0.9 / q;%1(hPa)での気圧変化
   %-0.15(hPa)で1(m)の変化率?
   %つまり-1(hPa)で20/3(mの変化率?)
   
        baro = u1 - u2;
        y_1 = baro * qq;
  
    y = y_1;
